simulink model "Assignement_Simulink_2"  (R2022b)
settings: Solver=ode8  StartTime=0.0  StopTime=20000  FixedStep=0.1  RelTol=1e-3
values from neighbouring files (symbols this model uses):
  a = 6.943e6    (= 6943000)    [Assignement_Script.m]
  A0 = eye(3,3)    [Assignement_Script.m]
  A1 = 0.02    [Assignement_Script.m]
  A2 = A1    (= 0.02)    [Assignement_Script.m]
  A3 = A1    (= 0.02)    [Assignement_Script.m]
  alpha_1 = 0.5    [Assignement_Script.m]
  alpha_2 = 0.5    [Assignement_Script.m]
  C_d = 2.1    [Assignement_Script.m]
  e = 0    [Assignement_Script.m]
  epsilon = 0.4093    [Assignement_Script.m]
  G = 6.6743e-11    [Assignement_Script.m]
  H0 = sqrt(g_10^2+g_11^2+h_11^2)    [Assignement_Script.m]
  i = 0.8    [Assignement_Script.m]
  I = 10^-2*diag([100.9,25.1,91.6])    [Assignement_Script.m]
  j_B = [0.01;0.05;0.01]    [Assignement_Script.m]
  k_d_detumbling = 0.01    [Assignement_Script.m]
  k_d_nadir = 0.012    [Assignement_Script.m]
  k_p_nadir = 0.012    [Assignement_Script.m]
  M_Earth = 5.972e24    (= 5.972e+24)    [Assignement_Script.m]
  n = sqrt(G*M_Earth/a^3)    [Assignement_Script.m]
  n_sun = 2*pi/T_sun    (= 1.99238499086e-07)    [Assignement_Script.m]
  omega_detumbling = [0; 0; n_SC]    [Assignement_Script.m]
  omega_nadir = omega_detumbling    [Assignement_Script.m]
  P = F_e/c    (= 4.52666666667e-06)    [Assignement_Script.m]
  position = 1e-2*[10,0,0;0,10,0;-10,0,0;0,-10,0;0,0,15;                                     0,0,-15;0,45,0;0,45,0;0,-45,0;0,-45,0]    [Assignement_Script.m]
  R_Earth = 6.378e6    (= 6378000)    [Assignement_Script.m]
  R_sun = 149597870000    [Assignement_Script.m]
  rhoD_vector = ones(10,1)*0.1    [Assignement_Script.m]
  rhoS_vector = ones(10,1)*0.5    [Assignement_Script.m]
  Surfaces_Matrix = [6e-2;6e-2;6e-2;6e-2;4e-2;4e-2;12e-2;                                                     12e-2;12e-2;12e-2]    [Assignement_Script.m]
  theta0 = 0    [Assignement_Script.m]
  Theta_m = deg2rad(11.5)    [Assignement_Script.m]
  time_detumbling = 500    [Assignement_Script.m]
  time_nadir_pointing = 500    [Assignement_Script.m]
  Versor_Surfaces_Matrix = [  1 , 0 ,-1 , 0 , 0 , 0 , 1 ,-1 , 1 ,-1 ... (first row only)    [Assignement_Script.m]
  w0 = [0.01;0.01;0.2]    [Assignement_Script.m]
  w_Earth = 7.29e-5    (= 7.29e-05)    [Assignement_Script.m]
undefined symbols (not defined in the file or in its folder): Gyroscope, HS, k_d_slew, k_i_tracking, k_p_slew, omega_slew, RW, SunSensor, time_slew
libraries: simulink_extras x14, sharedutil x12, vrlib x11, matrix_library x11, sharedtransform x2
(part 2 of 3)

== system Assignement_Simulink_2/  /Angular  Momentum ==
  Constant1 : Constant  Value=I
  Demux : Demux  Outputs=3
  Product1 : Product  Multiplication=Matrix(*)
  Square : Math  Operator=square
  Square Root : Sqrt
  Square1 : Math  Operator=square
  Square2 : Math  Operator=square
  Sum : Sum  Inputs=+++
  Out1 : Outport
  wires:
  [Omega] -> Product1/2
  Constant1/1 -> Product1/1
  Product1/1 -> Demux/1
  Square Root/1 -> Out1/1
  Demux/1 -> Square/1
  Demux/2 -> Square2/1
  Demux/3 -> Square1/1
  Square/1 -> Sum/1
  Square2/1 -> Sum/2
  Square1/1 -> Sum/3
  Sum/1 -> Square Root/1

== system Assignement_Simulink_2/  /Energy ==
  Constant1 : Constant  Value=I
  Gain : Gain  Gain=0.5
  Matrix Multiply : Product  Multiplication=Matrix(*)
  Matrix Multiply1 : Product  Multiplication=Matrix(*)
  Transpose : Math  Operator=transpose
  Out1 : Outport
  wires:
  Matrix Multiply1/1 -> Gain/1
  Matrix Multiply/1 -> Matrix Multiply1/1
  [Omega] -> Matrix Multiply1/2, Transpose/1
  Transpose/1 -> Matrix Multiply/1
  Gain/1 -> Out1/1
  Constant1/1 -> Matrix Multiply/2

== system Assignement_Simulink_2/ Magnetic Perturbance /Norm1 ==
  GPS Position2 : Inport
  Demux : Demux  Outputs=3
  Square : Math  Operator=square
  Square Root : Sqrt
  Square1 : Math  Operator=square
  Square2 : Math  Operator=square
  Sum : Sum  Inputs=+++
  Out1 : Outport
  wires:
  Demux/3 -> Square2/1
  Sum/1 -> Square Root/1
  Demux/1 -> Square/1
  Square1/1 -> Sum/2
  Demux/2 -> Square1/1
  GPS Position2/1 -> Demux/1
  Square2/1 -> Sum/3
  Square/1 -> Sum/1
  Square Root/1 -> Out1/1

== system Assignement_Simulink_2/ Magnetic Perturbance /m1 ==
  Clock : Clock
  Constant : Constant  Value=Theta_m
  Constant1 : Constant  Value=w_Earth
  Cos : Trigonometry  Operator=cos
  Cos1 : Trigonometry  Operator=cos
  Mux : Mux  Inputs=3
  Product : Product
  Product1 : Product
  Product2 : Product
  Sin : Trigonometry
  Sin1 : Trigonometry
  m : Outport
  wires:
  Constant/1 -> Sin/1, Cos1/1
  Clock/1 -> Product/2
  Constant1/1 -> Product/1
  Product/1 -> Sin1/1, Cos/1
  Sin/1 -> Product2/1, Product1/1
  Cos/1 -> Product1/2
  Sin1/1 -> Product2/2
  Product2/1 -> Mux/2
  Product1/1 -> Mux/1
  Cos1/1 -> Mux/3
  Mux/1 -> m/1

== system Assignement_Simulink_2/DCM/Anti-symmetric Matrix ==
  Omega : Inport
  Demux : Demux  Outputs=3
  Gain : Gain  Gain=[0,0,0;0,0,-1;0,1,0]
  Gain1 : Gain  Gain=[0,0,1;0,0,0;-1,0,0]
  Gain2 : Gain  Gain=[0,-1,0;1,0,0;0,0,0]
  Sum : Sum  Inputs=+++
  "[w]^" : Outport
  wires:
  Sum/1 -> "[w]^"/1
  Demux/1 -> Gain/1
  Gain/1 -> Sum/1
  Demux/3 -> Gain2/1
  Gain2/1 -> Sum/3
  Demux/2 -> Gain1/1
  Gain1/1 -> Sum/2
  Omega/1 -> Demux/1

== system Assignement_Simulink_2/DCM/Matrix determinant ==
  DCM : Inport
  Determinant of 3x3 Matrix : sharedutil/Determinant of 3x3 Matrix  aMode=aMode
      settings: LibrarySourceBlock=|
      | aerolibutil/Determinant of
      | 3x3 Matrix
  Determinant : Outport
  wires:
  Determinant of 3x3 Matrix/1 -> Determinant/1
  DCM/1 -> Determinant of 3x3 Matrix/1

== system Assignement_Simulink_2/DCM/Ortonormalizzation ==
  In1 : Inport
  Gain : Gain  Gain=1.5
  Gain1 : Gain  Gain=0.5
  Matrix Multiply : Product  Inputs=3  Multiplication=Matrix(*)
  Sum : Sum  Inputs=|+-
  Transpose : Math  Operator=transpose
  Output : Outport
  wires:
  Matrix Multiply/1 -> Gain1/1
  Gain/1 -> Sum/1
  In1/1 -> Matrix Multiply/3, Gain/1, Transpose/1, Matrix Multiply/1
  Gain1/1 -> Sum/2
  Transpose/1 -> Matrix Multiply/2
  Sum/1 -> Output/1

== system Assignement_Simulink_2/DCM/Perpendicularity ==
  DCM : Inport
  MATLAB Function2 : MATLAB Function  TreatAsAtomicUnit=on
  Perpendicularity flag : Outport
  wires:
  MATLAB Function2/1(perpendicularity_flag) -> Perpendicularity flag/1
  DCM/1 -> MATLAB Function2/1(DCM)

== system Assignement_Simulink_2/Drag Perturbances/Norm1 ==
  In1 : Inport
  Demux : Demux  Outputs=3
  Square : Math  Operator=square
  Square Root : Sqrt
  Square1 : Math  Operator=square
  Square2 : Math  Operator=square
  Sum : Sum  Inputs=+++
  Out1 : Outport
  wires:
  Demux/3 -> Square2/1
  Sum/1 -> Square Root/1
  Demux/1 -> Square/1
  Square1/1 -> Sum/2
  Demux/2 -> Square1/1
  In1/1 -> Demux/1
  Square2/1 -> Sum/3
  Square/1 -> Sum/1
  Square Root/1 -> Out1/1

== system Assignement_Simulink_2/Gravity Gradient Perturbation/Norm ==
  In1 : Inport
  Demux : Demux  Outputs=3
  Square : Math  Operator=square
  Square Root : Sqrt
  Square1 : Math  Operator=square
  Square2 : Math  Operator=square
  Sum : Sum  Inputs=+++
  Out1 : Outport
  wires:
  Demux/3 -> Square2/1
  Sum/1 -> Square Root/1
  Demux/1 -> Square/1
  Square1/1 -> Sum/2
  Demux/2 -> Square1/1
  In1/1 -> Demux/1
  Square2/1 -> Sum/3
  Square/1 -> Sum/1
  Square Root/1 -> Out1/1

== system Assignement_Simulink_2/Horizon sensor/Norm ==
  In1 : Inport
  Demux : Demux  Outputs=3
  Square : Math  Operator=square
  Square Root : Sqrt
  Square1 : Math  Operator=square
  Square2 : Math  Operator=square
  Sum : Sum  Inputs=+++
  Out1 : Outport
  wires:
  Demux/3 -> Square2/1
  Sum/1 -> Square Root/1
  Demux/1 -> Square/1
  Square1/1 -> Sum/2
  Demux/2 -> Square1/1
  In1/1 -> Demux/1
  Square2/1 -> Sum/3
  Square/1 -> Sum/1
  Square Root/1 -> Out1/1

== system Assignement_Simulink_2/Horizon sensor/Norm1 ==
  In1 : Inport
  Demux : Demux  Outputs=3
  Square : Math  Operator=square
  Square Root : Sqrt
  Square1 : Math  Operator=square
  Square2 : Math  Operator=square
  Sum : Sum  Inputs=+++
  Out1 : Outport
  wires:
  Demux/3 -> Square2/1
  Sum/1 -> Square Root/1
  Demux/1 -> Square/1
  Square1/1 -> Sum/2
  Demux/2 -> Square1/1
  In1/1 -> Demux/1
  Square2/1 -> Sum/3
  Square/1 -> Sum/1
  Square Root/1 -> Out1/1

== system Assignement_Simulink_2/Horizon sensor/Subsystem2 ==
  In1 : Inport
  Abs : Abs  SaturateOnIntegerOverflow=off
  Gain : Gain  Gain=1e-4
  Gain1 : Gain  Gain=1e-4
  Gain2 : Gain  Gain=1e-4
  Square : Math  Operator=square
  Sum : Sum  Inputs=++++
  Out1 : Outport
  wires:
  In1/1 -> Square/1, Abs/1, Gain/1, Sum/1
  Gain/1 -> Sum/2  "Scale"
  Gain1/1 -> Sum/3  "Assimmetry"
  Gain2/1 -> Sum/4  "Non-Linearity"
  Abs/1 -> Gain1/1
  Square/1 -> Gain2/1
  Sum/1 -> Out1/1

== system Assignement_Simulink_2/Horizon sensor/Subsystem3 ==
  In1 : Inport
  Abs : Abs  SaturateOnIntegerOverflow=off
  Gain : Gain  Gain=1e-4
  Gain1 : Gain  Gain=1e-4
  Gain2 : Gain  Gain=1e-4
  Square : Math  Operator=square
  Sum : Sum  Inputs=++++
  Out1 : Outport
  wires:
  In1/1 -> Sum/1, Square/1, Abs/1, Gain/1
  Gain/1 -> Sum/2  "Scale"
  Gain1/1 -> Sum/3  "Assimmetry"
  Gain2/1 -> Sum/4  "Non-Linearity"
  Abs/1 -> Gain1/1
  Square/1 -> Gain2/1
  Sum/1 -> Out1/1

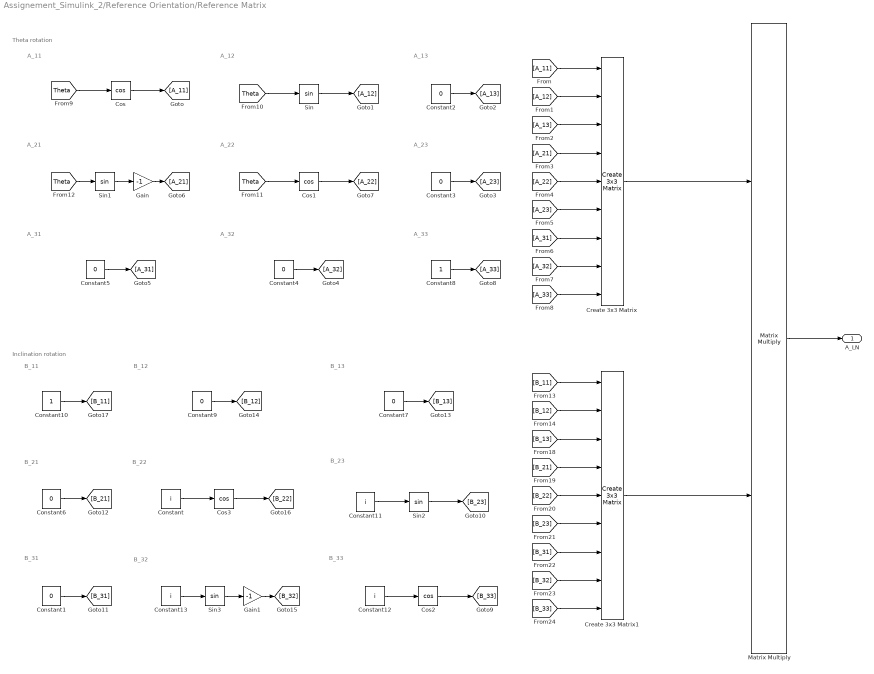
== system Assignement_Simulink_2/Reference Orientation/Reference Matrix ==
  note: Theta rotation
  note: A_11
  note: A_12
  note: A_13
  note: A_23
  note: A_33
  note: A_22
  note: A_21
  note: A_31
  note: A_32
  note: B_22
  note: B_33
  note: B_13
  note: B_23
  note: Inclination rotation
  note: B_21
  note: B_32
  note: B_11
  note: B_31
  note: B_12
  Constant{,11..13} (4 alike) : Constant  Value=i
  Constant{1..7,9} (8 alike) : Constant  Value=0
  Constant10 : Constant
  Constant8 : Constant
  Cos{,1..3} (4 alike) : Trigonometry  Operator=cos
  Create 3x3 Matrix : sharedutil/Create 3x3 Matrix  aMode=aMode
      settings: LibrarySourceBlock=aerolibutil/Create 3x3 Matrix
  Create 3x3 Matrix1 : sharedutil/Create 3x3 Matrix  aMode=aMode
      settings: LibrarySourceBlock=aerolibutil/Create 3x3 Matrix
  Gain : Gain  Gain=-1
  Gain1 : Gain  Gain=-1
  Matrix Multiply : Product  Multiplication=Matrix(*)
  Sin{,1..3} (4 alike) : Trigonometry
  A_LN : Outport
  wires:
  [Theta] -> Cos/1
  Cos/1 -> [A_11]
  Sin/1 -> [A_12]
  Constant2/1 -> [A_13]
  Constant3/1 -> [A_23]
  Constant4/1 -> [A_32]
  Constant5/1 -> [A_31]
  Sin1/1 -> Gain/1
  Cos1/1 -> [A_22]
  Constant8/1 -> [A_33]
  [A_11] -> Create 3x3 Matrix/1
  [A_12] -> Create 3x3 Matrix/2
  [A_13] -> Create 3x3 Matrix/3
  [A_21] -> Create 3x3 Matrix/4
  [A_22] -> Create 3x3 Matrix/5
  [A_23] -> Create 3x3 Matrix/6
  [A_31] -> Create 3x3 Matrix/7
  [A_32] -> Create 3x3 Matrix/8
  [A_33] -> Create 3x3 Matrix/9
  Create 3x3 Matrix/1 -> Matrix Multiply/1
  [Theta] -> Sin/1
  [Theta] -> Cos1/1
  [Theta] -> Sin1/1
  Gain/1 -> [A_21]
  Constant12/1 -> Cos2/1
  Constant13/1 -> Sin3/1
  Constant/1 -> Cos3/1
  [B_11] -> Create 3x3 Matrix1/1
  Constant6/1 -> [B_21]
  Constant10/1 -> [B_11]
  [B_12] -> Create 3x3 Matrix1/2
  Constant9/1 -> [B_12]
  Sin2/1 -> [B_23]
  Constant7/1 -> [B_13]
  Constant1/1 -> [B_31]
  Cos2/1 -> [B_33]
  Sin3/1 -> Gain1/1
  [B_23] -> Create 3x3 Matrix1/6
  [B_31] -> Create 3x3 Matrix1/7
  [B_33] -> Create 3x3 Matrix1/9
  Cos3/1 -> [B_22]
  Gain1/1 -> [B_32]
  [B_32] -> Create 3x3 Matrix1/8
  Create 3x3 Matrix1/1 -> Matrix Multiply/2
  [B_13] -> Create 3x3 Matrix1/3
  Constant11/1 -> Sin2/1
  [B_21] -> Create 3x3 Matrix1/4
  [B_22] -> Create 3x3 Matrix1/5
  Matrix Multiply/1 -> A_LN/1

== system Assignement_Simulink_2/Subsystem/Algebraic method ==
  HS_r_B : Inport
  SunSensor_s_B : Inport  Port=2
  Sun Position - Inerital frame : Inport  Port=3
  GPS Position : Inport  Port=4
  Enable : EnablePort
  Cross Product{,1..3} (4 alike) : matrix_library/Cross Product
  Determinant of 3x3 Matrix : sharedutil/Determinant of 3x3 Matrix  aMode=aMode
      settings: LibrarySourceBlock=|
      | aerolibutil/Determinant of
      | 3x3 Matrix
  Divide : Product  Inputs=*/
  Divide1 : Product  Inputs=*/
  Matrix Concatenate : Concatenate  NumInputs=3  Mode=Multidimensional array  ConcatenateDimension=2
  Matrix Concatenate1 : Concatenate  NumInputs=3  Mode=Multidimensional array  ConcatenateDimension=2
  Matrix Multiply : Product  Multiplication=Matrix(*)
  Norm : Subsystem
  Norm1 : Subsystem
  Normalize Vector{,1..3} (4 alike) : vrlib/Utilities/Normalize Vector  maxzero=0
  Scope : Scope
  Scope1 : Scope
  Transpose : Math  Operator=transpose
  Calculated DCM : Outport
  wires:
  Sun Position - Inerital frame/1 -> Cross Product2/2  "v1"
  Divide1/1 -> Scope1/1, Matrix Concatenate1/2, Cross Product3/2  "v2"
  Norm/1(norm) -> Divide/2
  Matrix Multiply/1 -> Calculated DCM/1
  Transpose/1 -> Matrix Multiply/2
  Norm1/1(norm) -> Divide1/2
  HS_r_B/1 -> Normalize Vector/1, Cross Product1/1, Cross Product/1
  Matrix Concatenate/1 -> Matrix Multiply/1
  Divide/1 -> Matrix Concatenate/2, Cross Product1/2  "s2"
  Determinant of 3x3 Matrix/1 -> Scope/1
  Cross Product/1 -> Norm/1(in), Divide/1
  Matrix Concatenate1/1 -> Determinant of 3x3 Matrix/1, Transpose/1
  Cross Product2/1 -> Norm1/1(in), Divide1/1
  SunSensor_s_B/1 -> Cross Product/2
  GPS Position/1 -> Normalize Vector2/1, Cross Product3/1, Cross Product2/1
  Normalize Vector/1 -> Matrix Concatenate/1  "s1"
  Cross Product1/1 -> Normalize Vector1/1  "s3"
  Normalize Vector1/1 -> Matrix Concatenate/3
  Normalize Vector2/1 -> Matrix Concatenate1/1  "s1"
  Normalize Vector3/1 -> Matrix Concatenate1/3  "s1"
  Cross Product3/1 -> Normalize Vector3/1  "v3"

== system Assignement_Simulink_2/Subsystem/Gyro propagation ==
  note: LOGIC
  note: TEST
  reset signal : Inport
  Gyro_Omega : Inport  Port=2
  Calculated DCM : Inport  Port=3
  Enable : EnablePort
  Anti-symmetric Matrix : Subsystem
  Gain1 : Gain  Gain=-1
  Integrator2 : Integrator  ExternalReset=level  InitialConditionSource=external
  Matrix Multiply1 : Product  Multiplication=Matrix(*)
  Matrix determinant : Subsystem
  Ortonormalizzation : Subsystem
  Perpendicularity : Subsystem
  Scope : Scope
  Scope1 : Scope
  Scope2 : Scope  NumInputPorts=2
  Gyro_DCM : Outport
  wires:
  Anti-symmetric Matrix/1("[w]^") -> Matrix Multiply1/1
  Gyro_Omega/1 -> Anti-symmetric Matrix/1(Omega)
  Ortonormalizzation/1(Output) -> Gyro_DCM/1, Perpendicularity/1(DCM), Matrix determinant/1(DCM), Matrix Multiply1/2
  Gain1/1 -> Integrator2/1
  Perpendicularity/1(Perpendicularity flag) -> Scope1/1
  Integrator2/1 -> Ortonormalizzation/1(In1)
  Matrix Multiply1/1 -> Gain1/1
  Matrix determinant/1(Determinant) -> Scope/1
  reset signal/1 -> Scope2/2, Integrator2/2
  Calculated DCM/1 -> Scope2/1, Integrator2/3

== system Assignement_Simulink_2/Subsystem1/Detumbling ==
  omega_gyro : Inport
  Enable : EnablePort
  Constant1 : Constant  Value=k_d_detumbling
  Constant2 : Constant  Value=omega_detumbling
  Product3 : Product
  Subtract : Sum  Inputs=+-
  M_detumbling : Outport  OutputWhenDisabled=reset  InitialOutput=[0 0 0]
  wires:
  Constant1/1 -> Product3/2
  Product3/1 -> M_detumbling/1
  Subtract/1 -> Product3/1
  Constant2/1 -> Subtract/2
  omega_gyro/1 -> Subtract/1

== system Assignement_Simulink_2/Subsystem1/Nadir Pointing ==
  Gyro_omega : Inport
  Extimated_DCM : Inport  Port=2
  A_LN : Inport  Port=3
  Enable : EnablePort
  Constant1 : Constant  Value=k_d_nadir
  Constant2 : Constant  Value=omega_nadir
  Constant3 : Constant  Value=k_p_nadir
  Product3 : Product
  Subtract : Sum  Inputs=+-
  Sum : Sum
  V operator : Subsystem
  M_nadir : Outport  OutputWhenDisabled=reset  InitialOutput=[0 0 0]
  wires:
  Constant1/1 -> Product3/2
  Subtract/1 -> Product3/1
  Constant2/1 -> Subtract/2
  Gyro_omega/1 -> Subtract/1
  A_LN/1 -> V operator/2(A_NL)
  Extimated_DCM/1 -> V operator/1(Extimated_DCM)
  Constant3/1 -> V operator/3(k_p_nadir)
  V operator/1(M_nadir) -> Sum/1
  Product3/1 -> Sum/2
  Sum/1 -> M_nadir/1

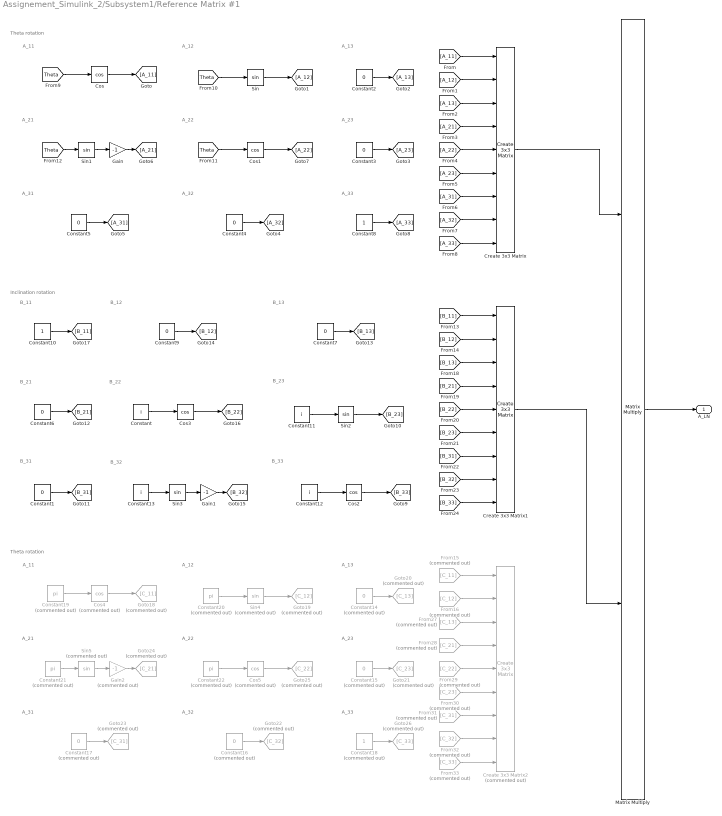
== system Assignement_Simulink_2/Subsystem1/Reference Matrix #1 ==
  note: Theta rotation
  note: A_11
  note: A_12
  note: A_13
  note: A_23
  note: A_33
  note: A_22
  note: A_21
  note: A_31
  note: A_32
  note: B_22
  note: B_33
  note: B_13
  note: B_23
  note: Inclination rotation
  note: B_21
  note: B_32
  note: B_11
  note: B_31
  note: B_12
  note: A_22
  note: A_12
  note: A_32
  note: A_11
  note: A_23
  note: A_13
  note: A_31
  note: A_21
  note: Theta rotation
  note: A_33
  Constant{,11..13} (4 alike) : Constant  Value=i
  Constant{1..7,9} (8 alike) : Constant  Value=0
  Constant10 : Constant
  Constant{14..17} (4 alike) : Constant  Commented=on  Value=0
  Constant18 : Constant  Commented=on
  Constant{19..22} (4 alike) : Constant  Commented=on  Value=pi
  Constant8 : Constant
  Cos{,1..3} (4 alike) : Trigonometry  Operator=cos
  Cos4 : Trigonometry  Commented=on  Operator=cos
  Cos5 : Trigonometry  Commented=on  Operator=cos
  Create 3x3 Matrix : sharedutil/Create 3x3 Matrix  aMode=aMode
      settings: LibrarySourceBlock=aerolibutil/Create 3x3 Matrix
  Create 3x3 Matrix1 : sharedutil/Create 3x3 Matrix  aMode=aMode
      settings: LibrarySourceBlock=aerolibutil/Create 3x3 Matrix
  Create 3x3 Matrix2 : sharedutil/Create 3x3 Matrix  Commented=on  aMode=aMode
      settings: LibrarySourceBlock=aerolibutil/Create 3x3 Matrix
  From15 : From  Commented=on  GotoTag=C_11
  From16 : From  Commented=on  GotoTag=C_12
  From27 : From  Commented=on  GotoTag=C_13
  From28 : From  Commented=on  GotoTag=C_21
  From29 : From  Commented=on  GotoTag=C_22
  From30 : From  Commented=on  GotoTag=C_23
  From31 : From  Commented=on  GotoTag=C_31
  From32 : From  Commented=on  GotoTag=C_32
  From33 : From  Commented=on  GotoTag=C_33
  Gain : Gain  Gain=-1
  Gain1 : Gain  Gain=-1
  Gain2 : Gain  Commented=on  Gain=-1
  Goto18 : Goto  Commented=on  GotoTag=C_11
  Goto19 : Goto  Commented=on  GotoTag=C_12
  Goto20 : Goto  Commented=on  GotoTag=C_13
  Goto21 : Goto  Commented=on  GotoTag=C_23
  Goto22 : Goto  Commented=on  GotoTag=C_32
  Goto23 : Goto  Commented=on  GotoTag=C_31
  Goto24 : Goto  Commented=on  GotoTag=C_21
  Goto25 : Goto  Commented=on  GotoTag=C_22
  Goto26 : Goto  Commented=on  GotoTag=C_33
  Matrix Multiply : Product  Multiplication=Matrix(*)
  Sin{,1..3} (4 alike) : Trigonometry
  Sin4 : Trigonometry  Commented=on
  Sin5 : Trigonometry  Commented=on
  A_LN : Outport
  wires:
  [Theta] -> Cos/1
  Cos/1 -> [A_11]
  Sin/1 -> [A_12]
  Constant2/1 -> [A_13]
  Constant3/1 -> [A_23]
  Constant4/1 -> [A_32]
  Constant5/1 -> [A_31]
  Sin1/1 -> Gain/1
  Cos1/1 -> [A_22]
  Constant8/1 -> [A_33]
  [A_11] -> Create 3x3 Matrix/1
  [A_12] -> Create 3x3 Matrix/2
  [A_13] -> Create 3x3 Matrix/3
  [A_21] -> Create 3x3 Matrix/4
  [A_22] -> Create 3x3 Matrix/5
  [A_23] -> Create 3x3 Matrix/6
  [A_31] -> Create 3x3 Matrix/7
  [A_32] -> Create 3x3 Matrix/8
  [A_33] -> Create 3x3 Matrix/9
  Create 3x3 Matrix/1 -> Matrix Multiply/1
  [Theta] -> Sin/1
  [Theta] -> Cos1/1
  [Theta] -> Sin1/1
  Gain/1 -> [A_21]
  Constant12/1 -> Cos2/1
  Constant13/1 -> Sin3/1
  Constant/1 -> Cos3/1
  [B_11] -> Create 3x3 Matrix1/1
  Constant6/1 -> [B_21]
  Constant10/1 -> [B_11]
  [B_12] -> Create 3x3 Matrix1/2
  Constant9/1 -> [B_12]
  Sin2/1 -> [B_23]
  Constant7/1 -> [B_13]
  Constant1/1 -> [B_31]
  Cos2/1 -> [B_33]
  Sin3/1 -> Gain1/1
  [B_23] -> Create 3x3 Matrix1/6
  [B_31] -> Create 3x3 Matrix1/7
  [B_33] -> Create 3x3 Matrix1/9
  Cos3/1 -> [B_22]
  Gain1/1 -> [B_32]
  [B_32] -> Create 3x3 Matrix1/8
  Create 3x3 Matrix1/1 -> Matrix Multiply/2
  [B_13] -> Create 3x3 Matrix1/3
  Constant11/1 -> Sin2/1
  [B_21] -> Create 3x3 Matrix1/4
  [B_22] -> Create 3x3 Matrix1/5
  Matrix Multiply/1 -> A_LN/1
  From15/1 -> Create 3x3 Matrix2/1
  From33/1 -> Create 3x3 Matrix2/9
  From16/1 -> Create 3x3 Matrix2/2
  Sin5/1 -> Gain2/1
  Constant21/1 -> Sin5/1
  From31/1 -> Create 3x3 Matrix2/7
  Gain2/1 -> Goto24/1
  Constant22/1 -> Cos5/1
  Constant20/1 -> Sin4/1
  From32/1 -> Create 3x3 Matrix2/8
  Constant19/1 -> Cos4/1
  Constant15/1 -> Goto21/1
  From30/1 -> Create 3x3 Matrix2/6
  From29/1 -> Create 3x3 Matrix2/5
  From27/1 -> Create 3x3 Matrix2/3
  Constant18/1 -> Goto26/1
  Cos4/1 -> Goto18/1
  Constant16/1 -> Goto22/1
  Cos5/1 -> Goto25/1
  From28/1 -> Create 3x3 Matrix2/4
  Sin4/1 -> Goto19/1
  Constant14/1 -> Goto20/1
  Constant17/1 -> Goto23/1

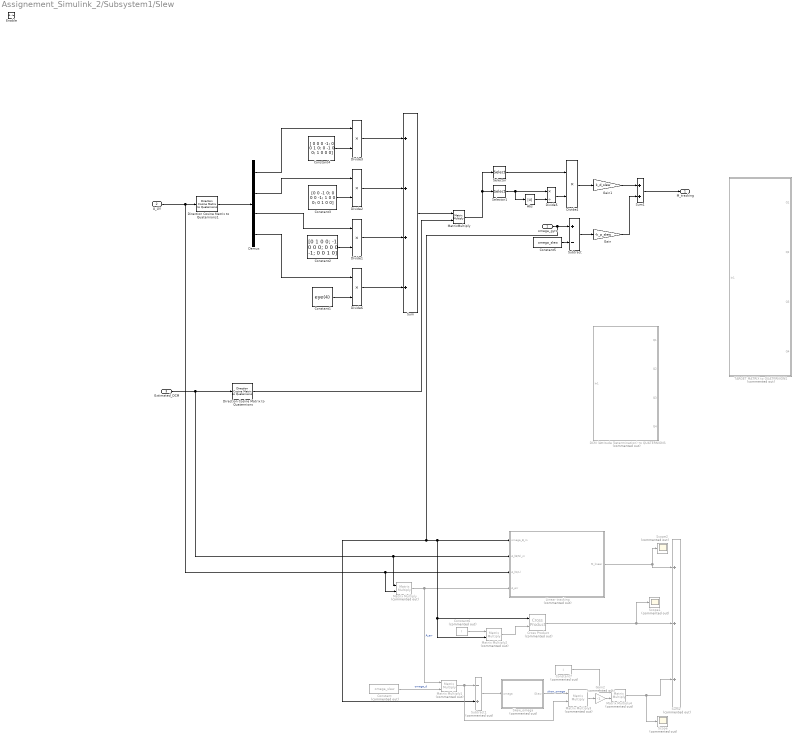
== system Assignement_Simulink_2/Subsystem1/Slew ==
  omega_gyro : Inport
  A_LN : Inport  Port=2
  Extimated_DCM : Inport  Port=3
  Enable : EnablePort
  Abs : Abs  SaturateOnIntegerOverflow=off
  Constant : Constant  Commented=on  Value=omega_slew
  Constant1 : Constant  Value=eye(4)
  Constant2 : Constant  Value=[0 1 0 0; -1 0 0 0; 0 0 0 -1; 0 0 1 0]
  Constant3 : Constant  Value=[0 0 -1 0; 0 0 0 -1; 1 0 0 0; 0 1 0 0]
  Constant4 : Constant  Value=[ 0 0 0 -1; 0 0 1 0; 0 -1 0 0; 1 0 0 0]
  Constant5 : Constant  Value=omega_slew
  Constant6 : Constant  Commented=on  Value=I
  Constant7 : Constant  Commented=on  Value=I
  Cross Product : matrix_library/Cross Product  Commented=on
  DCM (Attitude Determination) to QUATERNIONS : Subsystem  Commented=on
  Demux : Demux
  Direction Cosine Matrix to Quaternions : sharedtransform/Direction Cosine Matrix  to Quaternions  aMode=0  action=None  tolerance=eps(2)
      settings: LibrarySourceBlock=|
      | aerolibtransform2/Direction Cosine Matrix
      | to Quaternions
  Direction Cosine Matrix to Quaternions1 : sharedtransform/Direction Cosine Matrix  to Quaternions  aMode=0  action=None  tolerance=eps(2)
      settings: LibrarySourceBlock=|
      | aerolibtransform2/Direction Cosine Matrix
      | to Quaternions
  Divide{1..4,6} (5 alike) : Product  Inputs=**
  Divide5 : Product  Inputs=*/
  Gain : Gain  Gain=-k_p_slew
  Gain1 : Gain  Gain=k_d_slew
  Gain2 : Gain  Commented=on  Gain=-1
  Linear tracking : Subsystem  Commented=on
  Matrix Multiply{,1..4} (5 alike) : Product  Commented=on  Multiplication=Matrix(*)
  MatrixMultiply : Product  Multiplication=Matrix(*)
  Scope : Scope  Commented=on
  Scope1 : Scope  Commented=on
  Scope2 : Scope  Commented=on
  Selector : Selector  InputPortWidth=4  IndexOptions=Index vector (dialog)  Indices=[1 2 3]  OutputSizes=1
  Selector1 : Selector  InputPortWidth=4  IndexOptions=Index vector (dialog)  Indices=[4]  OutputSizes=1
  Skew_omega : Subsystem  Commented=on
  Subtract : Sum  Inputs=+-
  Subtract1 : Sum  Commented=on  Inputs=-+
  Sum : Sum  Inputs=++++
  Sum1 : Sum
  Sum2 : Sum  Commented=on  Inputs=+++
  TARGET MATRIX to QUATERNIONS : Subsystem  Commented=on
  M_tracking : Outport  OutputWhenDisabled=reset  InitialOutput=[0 0 0]
  wires:
  Gain1/1 -> Sum1/1
  Selector1/1 -> Abs/1, Divide5/1
  MatrixMultiply/1 -> Selector/1, Selector1/1
  Divide4/1 -> Gain1/1
  Abs/1 -> Divide5/2
  Divide5/1 -> Divide4/2
  Divide1/1 -> Sum/3
  Selector/1 -> Divide4/1
  Sum/1 -> MatrixMultiply/1
  Divide2/1 -> Sum/2
  Divide6/1 -> Sum/4
  Constant4/1 -> Divide3/2
  Divide3/1 -> Sum/1
  Constant3/1 -> Divide2/2
  Constant1/1 -> Divide6/2
  Direction Cosine Matrix to Quaternions/1 -> MatrixMultiply/2
  Subtract/1 -> Gain/1
  Constant2/1 -> Divide1/2
  Gain/1 -> Sum1/2
  Constant5/1 -> Subtract/2
  Linear tracking/1(M_linear) -> Sum2/1, Scope2/1
  Subtract1/1 -> Skew_omega/1(omega)
  Matrix Multiply2/1 -> Cross Product/2
  Matrix Multiply4/1 -> Sum2/3, Scope/1
  Cross Product/1 -> Scope1/1, Sum2/2
  Gain2/1 -> Matrix Multiply4/2
  Matrix Multiply/1 -> Matrix Multiply1/1, Linear tracking/4(A_err)  "A_err"
  Extimated_DCM/1 -> Direction Cosine Matrix to Quaternions/1, Matrix Multiply/1, Linear tracking/2(A_(B/N)_m)
  Constant7/1 -> Matrix Multiply4/1
  Matrix Multiply3/1 -> Gain2/1
  Skew_omega/1(Skew) -> Matrix Multiply3/1  "skew_omega"
  omega_gyro/1 -> Subtract1/2, Cross Product/1, Matrix Multiply2/2, Linear tracking/1(omega_B_m), Subtract/1
  A_LN/1 -> Direction Cosine Matrix to Quaternions1/1, Matrix Multiply/2, Linear tracking/3(A_(N/L))
  Constant/1 -> Matrix Multiply1/2  "omega_d"
  Constant6/1 -> Matrix Multiply2/1
  Matrix Multiply1/1 -> Matrix Multiply3/2, Subtract1/1
  Sum1/1 -> M_tracking/1
  Direction Cosine Matrix to Quaternions1/1 -> Demux/1
  Demux/1 -> Divide3/1
  Demux/2 -> Divide2/1
  Demux/3 -> Divide1/1
  Demux/4 -> Divide6/1

== system Assignement_Simulink_2/Subsystem1/Switch logic ==
  Clock : Clock
  Constant : Constant
  Constant1 : Constant  Value=-1
  Constant10 : Constant  Commented=on
  Constant8 : Constant  Value=-1
  Constant9 : Constant
  Gain : Gain  Gain=-1
  Gain4 : Gain  Commented=on  Gain=-1
  Switch : Switch  Criteria=u2 > Threshold  Threshold=time_detumbling  SaturateOnIntegerOverflow=off  InputSameDT=off
  Switch4 : Switch  Criteria=u2 > Threshold  Threshold=time_nadir_pointing  SaturateOnIntegerOverflow=off  InputSameDT=off
  Switch5 : Switch  Commented=on  Criteria=u2 > Threshold  Threshold=time_slew  SaturateOnIntegerOverflow=off  InputSameDT=off
  Detumbling : Outport
  Nadir : Outport  Port=2
  Slew : Outport  Port=3
  wires:
  Constant/1 -> Switch/1
  Constant1/1 -> Switch/3
  Switch/1 -> Gain/1
  Gain/1 -> Detumbling/1
  Switch4/1 -> Switch5/1, Nadir/1
  Constant10/1 -> Switch5/3
  Constant9/1 -> Switch4/1
  Switch5/1 -> Gain4/1
  Constant8/1 -> Switch4/3
  Clock/1 -> Switch5/2, Switch4/2, Switch/2
  Gain4/1 -> Slew/1

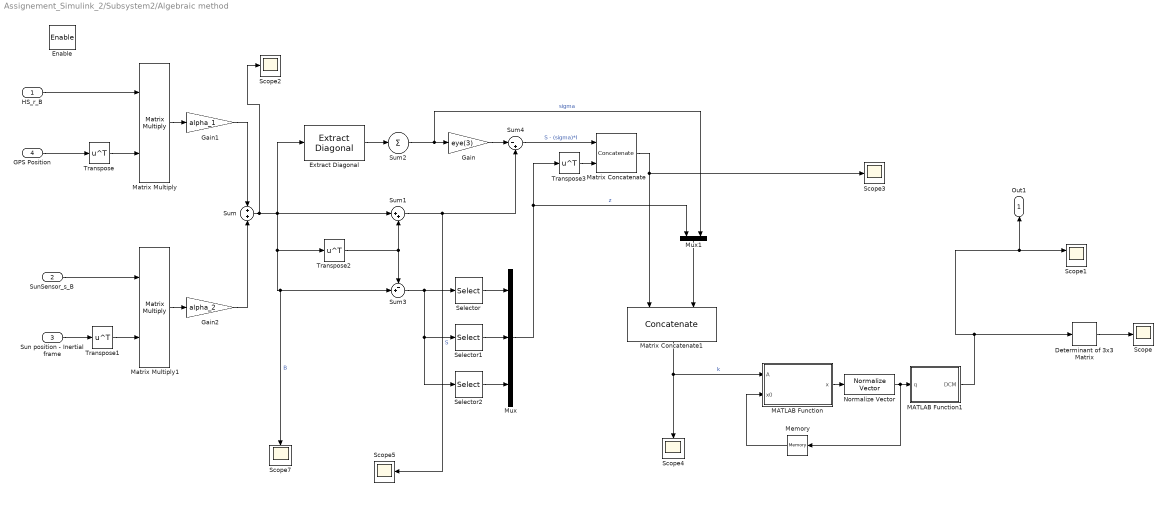
== system Assignement_Simulink_2/Subsystem2/Algebraic method ==
  HS_r_B : Inport
  SunSensor_s_B : Inport  Port=2
  Sun position - Inertial frame : Inport  Port=3
  GPS Position : Inport  Port=4
  Enable : EnablePort
  Determinant of 3x3 Matrix : sharedutil/Determinant of 3x3 Matrix  aMode=aMode
      settings: LibrarySourceBlock=|
      | aerolibutil/Determinant of
      | 3x3 Matrix
  Extract Diagonal : matrix_library/Extract Diagonal
      settings: LibrarySourceBlock=|
      | simulink/Matrix
      | Operations/Extract Diagonal
  Gain : Gain  Gain=eye(3)
  Gain1 : Gain  Gain=alpha_1
  Gain2 : Gain  Gain=alpha_2
  MATLAB Function : MATLAB Function  TreatAsAtomicUnit=on
  MATLAB Function1 : MATLAB Function  TreatAsAtomicUnit=on
  Matrix Concatenate : Concatenate  Mode=Multidimensional array
  Matrix Concatenate1 : Concatenate  Mode=Multidimensional array  ConcatenateDimension=2
  Matrix Multiply : Product  Multiplication=Matrix(*)
  Matrix Multiply1 : Product  Multiplication=Matrix(*)
  Memory : Memory  InitialCondition=[1;0;0;0]
  Mux : Mux  Inputs=3
  Mux1 : Mux  Inputs=2
  Normalize Vector : vrlib/Utilities/Normalize Vector  maxzero=0
  Scope{,2..5,7} (6 alike) : Scope
  Scope1 : Scope  NumInputPorts=2
  Selector : Selector  NumberOfDimensions=2  InputPortWidth=3  IndexOptions=Index vector (dialog),Index vector (dialog)  Indices=2,3  OutputSizes=1,1
  Selector1 : Selector  NumberOfDimensions=2  InputPortWidth=3  IndexOptions=Index vector (dialog),Index vector (dialog)  Indices=3,1  OutputSizes=1,1
  Selector2 : Selector  NumberOfDimensions=2  InputPortWidth=3  IndexOptions=Index vector (dialog),Index vector (dialog)  Indices=1,2  OutputSizes=1,1
  Sum : Sum
  Sum1 : Sum  Inputs=|++
  Sum2 : Sum  Inputs=+
  Sum3 : Sum  Inputs=-+|
  Sum4 : Sum  Inputs=|-+
  Transpose{,1..3} (4 alike) : Math  Operator=transpose
  Out1 : Outport
  wires:
  Transpose/1 -> Matrix Multiply/2
  Transpose1/1 -> Matrix Multiply1/2
  Matrix Multiply/1 -> Gain1/1
  Mux1/1 -> Matrix Concatenate1/2
  Sum/1 -> Extract Diagonal/1, Sum1/1, Transpose2/1, Scope7/1, Sum3/2, Scope2/1  "B"
  Mux/1 -> Mux1/1, Transpose3/1  "z"
  Sum2/1 -> Gain/1, Mux1/2  "sigma"
  Sum4/1 -> Matrix Concatenate/1  "S - (sigma)*I"
  GPS Position/1 -> Transpose/1
  Sum3/1 -> Selector/1, Selector1/1, Selector2/1
  HS_r_B/1 -> Matrix Multiply/1
  Transpose2/1 -> Sum3/1, Sum1/2
  Matrix Multiply1/1 -> Gain2/1
  Matrix Concatenate/1 -> Scope3/1, Matrix Concatenate1/1
  SunSensor_s_B/1 -> Matrix Multiply1/1
  Gain/1 -> Sum4/1
  Gain2/1 -> Sum/2
  Sum1/1 -> Sum4/2, Scope5/1  "S"
  Sun position - Inertial frame/1 -> Transpose1/1
  Selector1/1 -> Mux/2
  Matrix Concatenate1/1 -> Scope4/1, MATLAB Function/1(A)  "k"
  Extract Diagonal/1 -> Sum2/1
  Determinant of 3x3 Matrix/1 -> Scope/1
  Selector/1 -> Mux/1
  Selector2/1 -> Mux/3
  MATLAB Function1/1(DCM) -> Out1/1, Scope1/1, Determinant of 3x3 Matrix/1
  Transpose3/1 -> Matrix Concatenate/2
  Gain1/1 -> Sum/1
  MATLAB Function/1(x) -> Normalize Vector/1
  Memory/1 -> MATLAB Function/2(x0)
  Normalize Vector/1 -> Memory/1, MATLAB Function1/1(q)

== system Assignement_Simulink_2/Subsystem2/Gyro propagation ==
  note: TEST
  note: LOGIC
  reset signal : Inport
  Gyro_Omega : Inport  Port=2
  Calculated DCM : Inport  Port=3
  Enable : EnablePort
  Anti-symmetric Matrix : Subsystem
  Gain1 : Gain  Gain=-1
  Integrator2 : Integrator  ExternalReset=level  InitialConditionSource=external
  Matrix Multiply1 : Product  Multiplication=Matrix(*)
  Matrix determinant : Subsystem
  Ortonormalizzation : Subsystem
  Perpendicularity : Subsystem
  Scope : Scope
  Scope1 : Scope
  Scope2 : Scope  NumInputPorts=2
  Gyro_DCM : Outport
  wires:
  Calculated DCM/1 -> Integrator2/3, Scope2/1
  reset signal/1 -> Integrator2/2, Scope2/2
  Matrix determinant/1(Determinant) -> Scope/1
  Matrix Multiply1/1 -> Gain1/1
  Integrator2/1 -> Ortonormalizzation/1(In1)
  Perpendicularity/1(Perpendicularity flag) -> Scope1/1
  Gain1/1 -> Integrator2/1
  Ortonormalizzation/1(Output) -> Matrix Multiply1/2, Matrix determinant/1(DCM), Perpendicularity/1(DCM), Gyro_DCM/1
  Gyro_Omega/1 -> Anti-symmetric Matrix/1(Omega)
  Anti-symmetric Matrix/1("[w]^") -> Matrix Multiply1/1

== system Assignement_Simulink_2/Sun Sensor/Subsystem2 ==
  In1 : Inport
  Abs : Abs  SaturateOnIntegerOverflow=off
  Gain : Gain  Gain=1e-4
  Gain1 : Gain  Gain=1e-4
  Gain2 : Gain  Gain=1e-4
  Random Number : RandomNumber  Variance=0.1  SampleTime=0.1
  Square : Math  Operator=square
  Sum : Sum  Inputs=+++++
  Transfer Fcn : TransferFcn  Denominator=[1 1]
  Out1 : Outport
  wires:
  In1/1 -> Square/1, Abs/1, Gain/1, Sum/1
  Gain/1 -> Sum/2  "Scale"
  Gain1/1 -> Sum/3  "Assimmetry"
  Gain2/1 -> Sum/4  "Non-Linearity"
  Abs/1 -> Gain1/1
  Square/1 -> Gain2/1
  Sum/1 -> Out1/1
  Random Number/1 -> Transfer Fcn/1
  Transfer Fcn/1 -> Sum/5

== system Assignement_Simulink_2/Sun Sensor/Subsystem3 ==
  In1 : Inport
  Abs : Abs  SaturateOnIntegerOverflow=off
  Gain : Gain  Gain=1e-4
  Gain1 : Gain  Gain=1e-4
  Gain2 : Gain  Gain=1e-4
  Random Number : RandomNumber  Variance=0.1  SampleTime=0.1
  Square : Math  Operator=square
  Sum : Sum  Inputs=+++++
  Transfer Fcn : TransferFcn  Denominator=[1 1]
  Out1 : Outport
  wires:
  In1/1 -> Sum/1, Square/1, Abs/1, Gain/1
  Gain/1 -> Sum/2  "Scale"
  Gain1/1 -> Sum/3  "Assimmetry"
  Gain2/1 -> Sum/4  "Non-Linearity"
  Abs/1 -> Gain1/1
  Square/1 -> Gain2/1
  Sum/1 -> Out1/1
  Transfer Fcn/1 -> Sum/5
  Random Number/1 -> Transfer Fcn/1

== system Assignement_Simulink_2/Subsystem/Algebraic method/Norm ==
  in : Inport
  Dot Product1 : DotProduct  OutDataTypeStr=Inherit: Inherit via internal rule
  Sqrt : Sqrt
  norm : Outport
  wires:
  Sqrt/1 -> norm/1
  in/1 -> Dot Product1/2, Dot Product1/1
  Dot Product1/1 -> Sqrt/1

== system Assignement_Simulink_2/Subsystem/Algebraic method/Norm1 ==
  in : Inport
  Dot Product1 : DotProduct  OutDataTypeStr=Inherit: Inherit via internal rule
  Sqrt : Sqrt
  norm : Outport
  wires:
  Sqrt/1 -> norm/1
  in/1 -> Dot Product1/2, Dot Product1/1
  Dot Product1/1 -> Sqrt/1

== system Assignement_Simulink_2/Subsystem/Gyro propagation/Anti-symmetric Matrix ==
  Omega : Inport
  Demux : Demux  Outputs=3
  Gain : Gain  Gain=[0,0,0;0,0,-1;0,1,0]
  Gain1 : Gain  Gain=[0,0,1;0,0,0;-1,0,0]
  Gain2 : Gain  Gain=[0,-1,0;1,0,0;0,0,0]
  Sum : Sum  Inputs=+++
  "[w]^" : Outport
  wires:
  Sum/1 -> "[w]^"/1
  Demux/1 -> Gain/1
  Gain/1 -> Sum/1
  Demux/3 -> Gain2/1
  Gain2/1 -> Sum/3
  Demux/2 -> Gain1/1
  Gain1/1 -> Sum/2
  Omega/1 -> Demux/1

== system Assignement_Simulink_2/Subsystem/Gyro propagation/Matrix determinant ==
  DCM : Inport
  Determinant of 3x3 Matrix : sharedutil/Determinant of 3x3 Matrix  aMode=aMode
      settings: LibrarySourceBlock=|
      | aerolibutil/Determinant of
      | 3x3 Matrix
  Determinant : Outport
  wires:
  Determinant of 3x3 Matrix/1 -> Determinant/1
  DCM/1 -> Determinant of 3x3 Matrix/1

== system Assignement_Simulink_2/Subsystem/Gyro propagation/Ortonormalizzation ==
  In1 : Inport
  Gain : Gain  Gain=1.5
  Gain1 : Gain  Gain=0.5
  Matrix Multiply : Product  Inputs=3  Multiplication=Matrix(*)
  Sum : Sum  Inputs=|+-
  Transpose : Math  Operator=transpose
  Output : Outport
  wires:
  Matrix Multiply/1 -> Gain1/1
  Gain/1 -> Sum/1
  In1/1 -> Matrix Multiply/3, Gain/1, Transpose/1, Matrix Multiply/1
  Gain1/1 -> Sum/2
  Transpose/1 -> Matrix Multiply/2
  Sum/1 -> Output/1

== system Assignement_Simulink_2/Subsystem/Gyro propagation/Perpendicularity ==
  DCM : Inport
  MATLAB Function2 : MATLAB Function  TreatAsAtomicUnit=on
  Perpendicularity flag : Outport
  wires:
  MATLAB Function2/1(perpendicularity_flag) -> Perpendicularity flag/1
  DCM/1 -> MATLAB Function2/1(DCM)

== system Assignement_Simulink_2/Subsystem1/Nadir Pointing/V operator ==
  Extimated_DCM : Inport
  A_NL : Inport  Port=2
  k_p_nadir : Inport  Port=3
  -alpha_x : Selector  NumberOfDimensions=2  InputPortWidth=3  IndexOptions=Index vector (dialog),Index vector (dialog)  Indices=3,2  OutputSizes=1,1
  -alpha_y : Selector  NumberOfDimensions=2  InputPortWidth=3  IndexOptions=Index vector (dialog),Index vector (dialog)  Indices=1,3  OutputSizes=1,1
  -alpha_z : Selector  NumberOfDimensions=2  InputPortWidth=3  IndexOptions=Index vector (dialog),Index vector (dialog)  Indices=2,1  OutputSizes=1,1
  Gain2 : Gain  Gain=0.5
  Gain3 : Gain  Gain=0.5
  Gain4 : Gain  Gain=0.5
  Matrix Multiply : Product  Multiplication=Matrix(*)
  Mux : Mux  Inputs=3
  Product : Product
  Subtract1 : Sum  Inputs=+-
  Subtract2 : Sum  Inputs=+-
  Subtract3 : Sum  Inputs=+-
  alpha_x : Selector  NumberOfDimensions=2  InputPortWidth=3  IndexOptions=Index vector (dialog),Index vector (dialog)  Indices=2,3  OutputSizes=1,1
  alpha_y : Selector  NumberOfDimensions=2  InputPortWidth=3  IndexOptions=Index vector (dialog),Index vector (dialog)  Indices=3,1  OutputSizes=1,1
  alpha_z : Selector  NumberOfDimensions=2  InputPortWidth=3  IndexOptions=Index vector (dialog),Index vector (dialog)  Indices=1,2  OutputSizes=1,1
  M_nadir : Outport
  wires:
  Matrix Multiply/1 -> -alpha_x/1, alpha_x/1, -alpha_y/1, alpha_y/1, -alpha_z/1, alpha_z/1
  k_p_nadir/1 -> Product/2
  Gain2/1 -> Mux/1
  Subtract1/1 -> Gain2/1
  alpha_y/1 -> Subtract2/1
  Subtract3/1 -> Gain4/1
  alpha_x/1 -> Subtract1/1
  Subtract2/1 -> Gain3/1
  Gain3/1 -> Mux/2
  -alpha_z/1 -> Subtract3/2
  -alpha_y/1 -> Subtract2/2
  alpha_z/1 -> Subtract3/1
  Gain4/1 -> Mux/3
  -alpha_x/1 -> Subtract1/2
  Extimated_DCM/1 -> Matrix Multiply/1
  A_NL/1 -> Matrix Multiply/2
  Mux/1 -> Product/1
  Product/1 -> M_nadir/1

== system Assignement_Simulink_2/Subsystem1/Slew/DCM (Attitude Determination) to QUATERNIONS ==
  In1 : Inport
  A11 : Selector  NumberOfDimensions=2  InputPortWidth=1  IndexOptions=Index vector (dialog),Index vector (dialog)  Indices=1,1  OutputSizes=1,1
  A12 : Selector  NumberOfDimensions=2  InputPortWidth=3  IndexOptions=Index vector (dialog),Index vector (dialog)  Indices=1,2  OutputSizes=1,1
  A13 : Selector  NumberOfDimensions=2  InputPortWidth=3  IndexOptions=Index vector (dialog),Index vector (dialog)  Indices=1,3  OutputSizes=1,1
  A21 : Selector  NumberOfDimensions=2  InputPortWidth=3  IndexOptions=Index vector (dialog),Index vector (dialog)  Indices=2,1  OutputSizes=1,1
  A22 : Selector  NumberOfDimensions=2  InputPortWidth=3  IndexOptions=Index vector (dialog),Index vector (dialog)  Indices=2,2  OutputSizes=1,1
  A23 : Selector  NumberOfDimensions=2  InputPortWidth=3  IndexOptions=Index vector (dialog),Index vector (dialog)  Indices=2,3  OutputSizes=1,1
  A31 : Selector  NumberOfDimensions=2  InputPortWidth=3  IndexOptions=Index vector (dialog),Index vector (dialog)  Indices=3,1  OutputSizes=1,1
  A32 : Selector  NumberOfDimensions=2  InputPortWidth=3  IndexOptions=Index vector (dialog),Index vector (dialog)  Indices=3,2  OutputSizes=1,1
  A33 : Selector  NumberOfDimensions=2  InputPortWidth=3  IndexOptions=Index vector (dialog),Index vector (dialog)  Indices=3,3  OutputSizes=1,1
  Constant8 : Constant
  Divide6 : Product  Inputs=*/
  Divide7 : Product  Inputs=*/
  Divide8 : Product  Inputs=*/
  Gain2 : Gain  Gain=0.5
  Gain3 : Gain  Gain=1/4
  Gain4 : Gain  Gain=1/4
  Gain5 : Gain  Gain=1/4
  Sqrt : Sqrt
  Sum2 : Sum  Inputs=++++
  Sum3 : Sum  Inputs=+-
  Sum4 : Sum  Inputs=+-
  Sum5 : Sum  Inputs=+-
  Q1 : Outport
  Q2 : Outport  Port=2
  Q3 : Outport  Port=3
  Q4 : Outport  Port=4
  wires:
  Sum4/1 -> Gain4/1
  A33/1 -> Sum2/4
  Sum5/1 -> Gain5/1
  A32/1 -> Sum3/2
  Gain2/1 -> Q4/1, Divide6/2, Divide7/2, Divide8/2
  A12/1 -> Sum5/1
  Gain3/1 -> Divide6/1
  Divide8/1 -> Q3/1
  Sum2/1 -> Sqrt/1
  In1/1 -> A23/1, A32/1, A31/1, A13/1, A12/1, A21/1, A33/1, A22/1, A11/1
  Constant8/1 -> Sum2/1
  Gain5/1 -> Divide8/1
  A23/1 -> Sum3/1
  Gain4/1 -> Divide7/1
  A22/1 -> Sum2/3
  Divide6/1 -> Q1/1
  Sqrt/1 -> Gain2/1
  A11/1 -> Sum2/2
  A21/1 -> Sum5/2
  Sum3/1 -> Gain3/1
  A31/1 -> Sum4/1
  A13/1 -> Sum4/2
  Divide7/1 -> Q2/1

== system Assignement_Simulink_2/Subsystem1/Slew/Linear tracking ==
  omega_B_m : Inport
  A_(B/N)_m : Inport  Port=2
  A_(N/L) : Inport  Port=3
  A_err : Inport  Port=4
  Constant1 : Constant  Value=omega_slew
  Constant2 : Constant  Commented=on  Value=k_i_tracking
  Delay : Delay  Commented=on  DelayLength=1
  Gain : Gain  Gain=[1 1 1]*k_d_slew
  Gain1 : Gain  Gain=-1
  Gain2 : Gain  Gain=[1 1 1]*k_p_slew
  Gain3 : Gain  Gain=-1
  Gain4 : Gain  Commented=on  Gain=-1
  IC : InitialCondition  Commented=on  Value=[0,0,0]
  Matrix Multiply : Product  Commented=on
  Matrix Multiply1 : Product  Multiplication=Matrix(*)
  Scope : Scope  Commented=on
  Subtract : Sum  Inputs=+-
  Sum : Sum  Inputs=+++
  Sum1 : Sum  Commented=on  Inputs=|++
  V operator : Subsystem
  V operator2 : Subsystem  Commented=on
  M_linear : Outport
  wires:
  A_(N/L)/1 -> V operator/2(A_(N/L)), V operator2/2(A_(N/L))
  Constant1/1 -> Matrix Multiply1/2
  Subtract/1 -> Gain/1
  A_(B/N)_m/1 -> V operator/1(A_m), V operator2/1(A_m)
  omega_B_m/1 -> Subtract/1
  A_err/1 -> Matrix Multiply1/1  "A_err"
  Matrix Multiply1/1 -> Subtract/2
  Gain/1 -> Gain1/1
  V operator/1(M2) -> Gain2/1
  Gain1/1 -> Sum/1
  Sum/1 -> M_linear/1
  Sum1/1 -> Matrix Multiply/1, Delay/1
  IC/1 -> Sum1/1
  Gain2/1 -> Gain3/1
  Gain3/1 -> Sum/2
  V operator2/1(err) -> IC/1
  Constant2/1 -> Matrix Multiply/2
  Matrix Multiply/1 -> Gain4/1
  Gain4/1 -> Sum/3, Scope/1
  Delay/1 -> Sum1/2

== system Assignement_Simulink_2/Subsystem1/Slew/Skew_omega ==
  omega : Inport
  0 : Constant  Value=0
  Create 3x3 Matrix : sharedutil/Create 3x3 Matrix  aMode=aMode
  Demux : Demux  Outputs=3
  Gain : Gain  Gain=-1
  Gain1 : Gain  Gain=-1
  Gain2 : Gain  Gain=-1
  Skew : Outport
  wires:
  Demux/1 -> Create 3x3 Matrix/8, Gain1/1  "omega_x"
  0/1 -> Create 3x3 Matrix/5, Create 3x3 Matrix/1, Create 3x3 Matrix/9  "0"
  Gain2/1 -> Create 3x3 Matrix/7
  Gain1/1 -> Create 3x3 Matrix/6
  Demux/2 -> Gain2/1, Create 3x3 Matrix/3
  Demux/3 -> Gain/1, Create 3x3 Matrix/4
  Gain/1 -> Create 3x3 Matrix/2
  omega/1 -> Demux/1
  Create 3x3 Matrix/1 -> Skew/1

== system Assignement_Simulink_2/Subsystem1/Slew/TARGET MATRIX to QUATERNIONS ==
  In1 : Inport
  A11 : Selector  NumberOfDimensions=2  InputPortWidth=1  IndexOptions=Index vector (dialog),Index vector (dialog)  Indices=1,1  OutputSizes=1,1
  A12 : Selector  NumberOfDimensions=2  InputPortWidth=3  IndexOptions=Index vector (dialog),Index vector (dialog)  Indices=1,2  OutputSizes=1,1
  A13 : Selector  NumberOfDimensions=2  InputPortWidth=3  IndexOptions=Index vector (dialog),Index vector (dialog)  Indices=1,3  OutputSizes=1,1
  A21 : Selector  NumberOfDimensions=2  InputPortWidth=3  IndexOptions=Index vector (dialog),Index vector (dialog)  Indices=2,1  OutputSizes=1,1
  A22 : Selector  NumberOfDimensions=2  InputPortWidth=3  IndexOptions=Index vector (dialog),Index vector (dialog)  Indices=2,2  OutputSizes=1,1
  A23 : Selector  NumberOfDimensions=2  InputPortWidth=3  IndexOptions=Index vector (dialog),Index vector (dialog)  Indices=2,3  OutputSizes=1,1
  A31 : Selector  NumberOfDimensions=2  InputPortWidth=3  IndexOptions=Index vector (dialog),Index vector (dialog)  Indices=3,1  OutputSizes=1,1
  A32 : Selector  NumberOfDimensions=2  InputPortWidth=3  IndexOptions=Index vector (dialog),Index vector (dialog)  Indices=3,2  OutputSizes=1,1
  A33 : Selector  NumberOfDimensions=2  InputPortWidth=3  IndexOptions=Index vector (dialog),Index vector (dialog)  Indices=3,3  OutputSizes=1,1
  Constant8 : Constant
  Divide6 : Product  Inputs=*/
  Divide7 : Product  Inputs=*/
  Divide8 : Product  Inputs=*/
  Gain2 : Gain  Gain=0.5
  Gain3 : Gain  Gain=1/4
  Gain4 : Gain  Gain=1/4
  Gain5 : Gain  Gain=1/4
  Sqrt : Sqrt
  Sum2 : Sum  Inputs=++++
  Sum3 : Sum  Inputs=+-
  Sum4 : Sum  Inputs=+-
  Sum5 : Sum  Inputs=+-
  Q1 : Outport
  Q2 : Outport  Port=2
  Q3 : Outport  Port=3
  Q4 : Outport  Port=4
  wires:
  Sum4/1 -> Gain4/1
  A33/1 -> Sum2/4
  Sum5/1 -> Gain5/1
  A32/1 -> Sum3/2
  Gain2/1 -> Q4/1, Divide6/2, Divide7/2, Divide8/2
  A12/1 -> Sum5/1
  Gain3/1 -> Divide6/1
  Divide8/1 -> Q3/1
  Sum2/1 -> Sqrt/1
  In1/1 -> A23/1, A32/1, A31/1, A13/1, A12/1, A21/1, A33/1, A22/1, A11/1
  Constant8/1 -> Sum2/1
  Gain5/1 -> Divide8/1
  A23/1 -> Sum3/1
  Gain4/1 -> Divide7/1
  A22/1 -> Sum2/3
  Divide6/1 -> Q1/1
  Sqrt/1 -> Gain2/1
  A11/1 -> Sum2/2
  A21/1 -> Sum5/2
  Sum3/1 -> Gain3/1
  A31/1 -> Sum4/1
  A13/1 -> Sum4/2
  Divide7/1 -> Q2/1

== system Assignement_Simulink_2/Subsystem2/Gyro propagation/Anti-symmetric Matrix ==
  Omega : Inport
  Demux : Demux  Outputs=3
  Gain : Gain  Gain=[0,0,0;0,0,-1;0,1,0]
  Gain1 : Gain  Gain=[0,0,1;0,0,0;-1,0,0]
  Gain2 : Gain  Gain=[0,-1,0;1,0,0;0,0,0]
  Sum : Sum  Inputs=+++
  "[w]^" : Outport
  wires:
  Omega/1 -> Demux/1
  Gain1/1 -> Sum/2
  Demux/2 -> Gain1/1
  Gain2/1 -> Sum/3
  Demux/3 -> Gain2/1
  Gain/1 -> Sum/1
  Demux/1 -> Gain/1
  Sum/1 -> "[w]^"/1

== system Assignement_Simulink_2/Subsystem2/Gyro propagation/Matrix determinant ==
  DCM : Inport
  Determinant of 3x3 Matrix : sharedutil/Determinant of 3x3 Matrix  aMode=aMode
      settings: LibrarySourceBlock=|
      | aerolibutil/Determinant of
      | 3x3 Matrix
  Determinant : Outport
  wires:
  DCM/1 -> Determinant of 3x3 Matrix/1
  Determinant of 3x3 Matrix/1 -> Determinant/1

== system Assignement_Simulink_2/Subsystem2/Gyro propagation/Ortonormalizzation ==
  In1 : Inport
  Gain : Gain  Gain=1.5
  Gain1 : Gain  Gain=0.5
  Matrix Multiply : Product  Inputs=3  Multiplication=Matrix(*)
  Sum : Sum  Inputs=|+-
  Transpose : Math  Operator=transpose
  Output : Outport
  wires:
  Sum/1 -> Output/1
  Transpose/1 -> Matrix Multiply/2
  Gain1/1 -> Sum/2
  In1/1 -> Matrix Multiply/1, Transpose/1, Gain/1, Matrix Multiply/3
  Gain/1 -> Sum/1
  Matrix Multiply/1 -> Gain1/1

== system Assignement_Simulink_2/Subsystem2/Gyro propagation/Perpendicularity ==
  DCM : Inport
  MATLAB Function2 : MATLAB Function  TreatAsAtomicUnit=on
  Perpendicularity flag : Outport
  wires:
  DCM/1 -> MATLAB Function2/1(DCM)
  MATLAB Function2/1(perpendicularity_flag) -> Perpendicularity flag/1

== system Assignement_Simulink_2/Subsystem1/Slew/Linear tracking/V operator ==
  A_m : Inport
  A_(N/L) : Inport  Port=2
  -alpha_x : Selector  NumberOfDimensions=2  InputPortWidth=3  IndexOptions=Index vector (dialog),Index vector (dialog)  Indices=3,2  OutputSizes=1,1
  -alpha_y : Selector  NumberOfDimensions=2  InputPortWidth=3  IndexOptions=Index vector (dialog),Index vector (dialog)  Indices=1,3  OutputSizes=1,1
  -alpha_z : Selector  NumberOfDimensions=2  InputPortWidth=3  IndexOptions=Index vector (dialog),Index vector (dialog)  Indices=2,1  OutputSizes=1,1
  Gain2 : Gain  Gain=0.5
  Gain3 : Gain  Gain=0.5
  Gain4 : Gain  Gain=0.5
  Matrix Multiply : Product  Multiplication=Matrix(*)
  Mux : Mux  Inputs=3
  Subtract1 : Sum  Inputs=+-
  Subtract2 : Sum  Inputs=+-
  Subtract3 : Sum  Inputs=+-
  alpha_x : Selector  NumberOfDimensions=2  InputPortWidth=3  IndexOptions=Index vector (dialog),Index vector (dialog)  Indices=2,3  OutputSizes=1,1
  alpha_y : Selector  NumberOfDimensions=2  InputPortWidth=3  IndexOptions=Index vector (dialog),Index vector (dialog)  Indices=3,1  OutputSizes=1,1
  alpha_z : Selector  NumberOfDimensions=2  InputPortWidth=3  IndexOptions=Index vector (dialog),Index vector (dialog)  Indices=1,2  OutputSizes=1,1
  M2 : Outport
  wires:
  Matrix Multiply/1 -> -alpha_x/1, alpha_x/1, -alpha_y/1, alpha_y/1, -alpha_z/1, alpha_z/1
  Mux/1 -> M2/1
  Subtract1/1 -> Gain2/1
  alpha_y/1 -> Subtract2/1
  Subtract3/1 -> Gain4/1
  alpha_x/1 -> Subtract1/1
  Subtract2/1 -> Gain3/1
  Gain2/1 -> Mux/1
  Gain3/1 -> Mux/2
  -alpha_z/1 -> Subtract3/2
  -alpha_y/1 -> Subtract2/2
  alpha_z/1 -> Subtract3/1
  -alpha_x/1 -> Subtract1/2
  A_m/1 -> Matrix Multiply/1
  A_(N/L)/1 -> Matrix Multiply/2
  Gain4/1 -> Mux/3

== system Assignement_Simulink_2/Subsystem1/Slew/Linear tracking/V operator2 ==
  A_m : Inport
  A_(N/L) : Inport  Port=2
  -alpha_x : Selector  NumberOfDimensions=2  InputPortWidth=3  IndexOptions=Index vector (dialog),Index vector (dialog)  Indices=3,2  OutputSizes=1,1
  -alpha_y : Selector  NumberOfDimensions=2  InputPortWidth=3  IndexOptions=Index vector (dialog),Index vector (dialog)  Indices=1,3  OutputSizes=1,1
  -alpha_z : Selector  NumberOfDimensions=2  InputPortWidth=3  IndexOptions=Index vector (dialog),Index vector (dialog)  Indices=2,1  OutputSizes=1,1
  Gain2 : Gain  Gain=0.5
  Gain3 : Gain  Gain=0.5
  Gain4 : Gain  Gain=0.5
  Matrix Multiply : Product  Multiplication=Matrix(*)
  Mux : Mux  Inputs=3
  Subtract1 : Sum  Inputs=+-
  Subtract2 : Sum  Inputs=+-
  Subtract3 : Sum  Inputs=+-
  alpha_x : Selector  NumberOfDimensions=2  InputPortWidth=3  IndexOptions=Index vector (dialog),Index vector (dialog)  Indices=2,3  OutputSizes=1,1
  alpha_y : Selector  NumberOfDimensions=2  InputPortWidth=3  IndexOptions=Index vector (dialog),Index vector (dialog)  Indices=3,1  OutputSizes=1,1
  alpha_z : Selector  NumberOfDimensions=2  InputPortWidth=3  IndexOptions=Index vector (dialog),Index vector (dialog)  Indices=1,2  OutputSizes=1,1
  err : Outport
  wires:
  Matrix Multiply/1 -> -alpha_x/1, alpha_x/1, -alpha_y/1, alpha_y/1, -alpha_z/1, alpha_z/1
  Mux/1 -> err/1
  Subtract1/1 -> Gain2/1
  alpha_y/1 -> Subtract2/1
  Subtract3/1 -> Gain4/1
  alpha_x/1 -> Subtract1/1
  Subtract2/1 -> Gain3/1
  Gain2/1 -> Mux/1
  Gain3/1 -> Mux/2
  -alpha_z/1 -> Subtract3/2
  -alpha_y/1 -> Subtract2/2
  alpha_z/1 -> Subtract3/1
  -alpha_x/1 -> Subtract1/2
  A_m/1 -> Matrix Multiply/1
  A_(N/L)/1 -> Matrix Multiply/2
  Gain4/1 -> Mux/3

== matlab function Assignement_Simulink_2/Wabba Problem   /MATLAB Function1 ==
  data: q input; DCM output
function DCM = fcn(q)

q1 = q(1);
q2 = q(2);
q3 = q(3);
q4 = q(4);

DCM = [q1^2-q2^2-q3^2+q4^2, 2*(q1*q2+q3*q4), 2*(q1*q3-q2*q4);
        2*(q1*q2-q3*q4), -q1^2+q2^2-q3^2+q4^2, 2*(q2*q3+q1*q4);
        2*(q1*q3+q2*q4), 2*(q2*q3-q1*q4), -q1^2-q2^2+q3^2+q4^2];

end

== matlab function Assignement_Simulink_2/Wabba Problem   /MATLAB Function ==
  data: A input; x output; x0 input
function x  = eigpower_io(A, x0)
tol = 1e-4;
y = x0/norm(x0);  % approssimazione autovettore
lambda = y'*A*y; % approssiamzione autovalore
lambda_ex = lambda;
x = A*y;
y = x/norm(x);
lambda = y'*A*y;

while (abs(lambda-lambda_ex)/abs(lambda))>tol
    lambda_ex = lambda;
    x = A*y;
    y = x/norm(x);
    lambda = y'*A*y;
end

end

== matlab function Assignement_Simulink_2/Subsystem/Gyro propagation/Perpendicularity/MATLAB Function2 ==
  data: DCM input; perpendicularity_flag output
function perpendicularity_flag = fcn(DCM)
    

perpendicularity_flag =zeros(3,1);

    x   = DCM(1,:);
    y   = DCM(2,:);
    z   = DCM(3,:);

    perpendicularity_flag(1)=dot(x,y);
    perpendicularity_flag(2)=dot(x,z);
    perpendicularity_flag(3)=dot(z,y);

end

== matlab function Assignement_Simulink_2/DCM/Perpendicularity/MATLAB Function2 ==
  data: DCM input; perpendicularity_flag output
function perpendicularity_flag = fcn(DCM)
    

perpendicularity_flag =zeros(3,1);

    x   = DCM(1,:);
    y   = DCM(2,:);
    z   = DCM(3,:);

    perpendicularity_flag(1)=dot(x,y);
    perpendicularity_flag(2)=dot(x,z);
    perpendicularity_flag(3)=dot(z,y);

end

== matlab function Assignement_Simulink_2/Drag Perturbances/Air density relation ==
  data: r_N input; R_Earth input; rho output
function rho = density_calculator(r_N, R_Earth)
% Exponential model for computing density

h = (norm(r_N') - R_Earth)/1e+3;


H = 0;
h0 = 0;
rho_0 = 0; 

if h > 200 && h <= 250
    H = 38.5;
    h0 = 200;
    rho_0 = 2.780e-10;
elseif h > 250 && h <= 300
    H = 46.9;
    h0 = 250;
    rho_0 = 7.248e-11;
elseif h > 300 && h <= 350
    H = 52.5;
    h0 = 300;
    rho_0 = 2.418e-11;
elseif h > 350 && h <= 400
    H = 56.4;
    h0 = 350;
    rho_0 = 9.158e-12;
elseif h > 400 && h <= 450
    H = 59.4;
    h0 = 400;
    rho_0 = 3.725e-12;
elseif h > 450 && h <= 500
    H = 62.2;
    h0 = 450;
    rho_0 = 1.585e-12;
elseif h > 500 && h <= 600
    H = 65.8;
    h0 = 500;
    rho_0 = 6.967e-13;
elseif h > 600 && h <= 700
    H = 79.0;
    h0 = 600;
    rho_0 = 1.454e-13;
elseif h > 700 && h <= 800
    H = 109.0;
    h0 = 700;
    rho_0 = 3.614e-14;
elseif h > 800 && h <= 900
    H = 164.0;
    h0 = 800;
    rho_0 = 1.170e-14;
elseif h > 900 && h < 1000
    H = 225.0;
    h0 = 900;
    rho_0 = 5.245e-15;
elseif h > 1000 
    H = 260.0;
    h0 = 1000;
    rho_0 = 3.019e-15;
end

rho = rho_0*exp(-(h-h0)/H)*1e+20;
